simulink library "Batteries"  (R2024b)
settings: Solver=VariableStepAuto  StartTime=0.0  StopTime=10.0  RelTol=1e-3
undefined symbols (not defined in the file or in its folder): battery_builder_rtmsupport, gcbh
libraries: nesl_utility x25, Batteries_lib x25
(part 2 of 2)

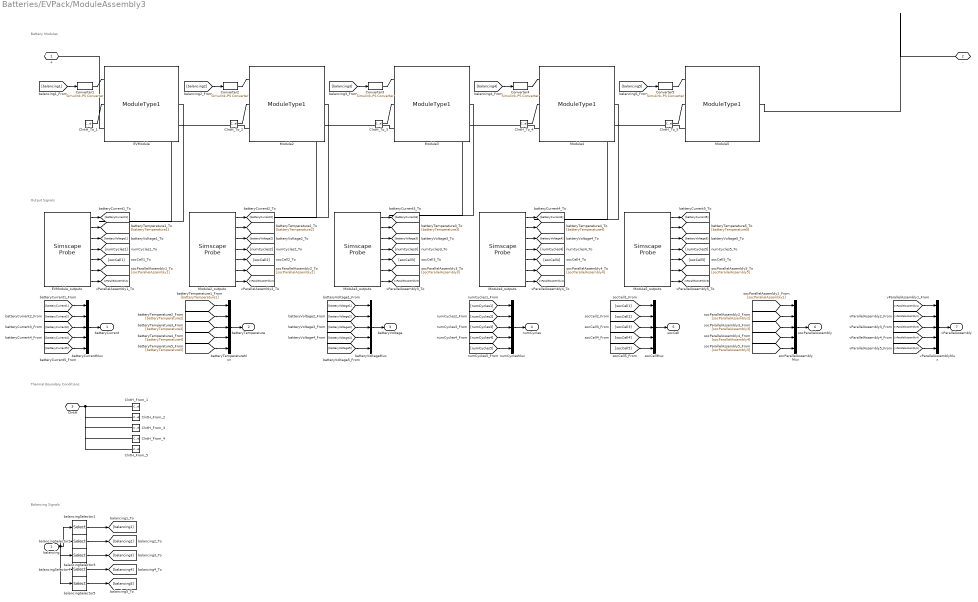
== system Batteries/EVPack/ModuleAssembly3 ==
  note: Balancing Signals
  note: Thermal Boundary Conditions
  note: Output Signals
  note: Battery Modules
  balancing : Inport  PortDimensions=25
  ClntH_From_1 : ConnectionLabel  Label=clntH_1
  ClntH_From_2 : ConnectionLabel  Label=clntH_2
  ClntH_From_3 : ConnectionLabel  Label=clntH_3
  ClntH_From_4 : ConnectionLabel  Label=clntH_4
  ClntH_From_5 : ConnectionLabel  Label=clntH_5
  ClntH_To_1 : ConnectionLabel  Label=clntH_1
  ClntH_To_2 : ConnectionLabel  Label=clntH_2
  ClntH_To_3 : ConnectionLabel  Label=clntH_3
  ClntH_To_4 : ConnectionLabel  Label=clntH_4
  ClntH_To_5 : ConnectionLabel  Label=clntH_5
  Converter{1..5} (5 alike) : nesl_utility/Simulink-PS Converter  PhysicalDomain=network_engine_domain  SubClassName=ps_input  LeftPortType=input  RightPortType=output  PseudoPeriodic=off  Frequencies=[]  NoiseDistribution=none  NoiseParameters=[]  Unit=1  AffineConversion=off  FilteringAndDerivatives=provide  SimscapeFilterOrder=1  InputFilterTimeConstant=0.001  UdotUserProvided=0
  EVModule : Batteries_lib/Modules/ModuleType1  BatteryCapacityCell=27 A*hr  ExtrapolationMethodCell=simscape.enum.extrapolation.nearest  SOCBreakpointsCell=[0, .1, .25, .5, .75, .9, 1]  TemperatureBreakpointsCell=[278, 293, 313] K  OpenCircuitVoltageThermalCell=[3.49, 3.5, 3.51; 3.55, 3.57, 3.56; 3.62, 3.63, 3.64; 3.71, 3.71, 3.72; 3.91, 3.93, 3.94; 4.07, 4.08, 4.08; 4.19, 4.19, 4.19] V  VoltageRangeCell=[0, inf] V  ResistanceSOCBreakpointsCell=[0, .1, .25, .5, .75, .9, 1]  ResistanceTemperatureBreakpointsCell=[278, 293, 313] K  R0ThermalCell=[.0117, .0085, .009; .011, .0085, .009; .0114, .0087, .0092; .0107, .0082, .0088; .0107, .0083, .0091; .0113, .0085, .0089; .0116, .0085, .0089] Ohm  BatteryThermalMassCell=100 J/K  CoolantResistance=1.2 K/W  CellBalancingClosedResistance=0.01 Ohm  CellBalancingOpenConductance=1e-8 1/Ohm  CellBalancingThreshold=0.5  CellBalancingResistance=50 Ohm  P=4  S=5  socCell_specify=off  socCell_priority=High  socCell=1  socCell_nominal_specify=off  socCell_nominal_value=1  socCell_nominal_unit=1  numCycles_specify=off  numCycles_priority=High  numCycles=0  numCycles_nominal_specify=off  numCycles_nominal_value=1  numCycles_nominal_unit=1  batteryVoltage_specify=off  batteryVoltage_priority=None  batteryVoltage=0 V  batteryVoltage_nominal_specify=off  batteryVoltage_nominal_value=1  batteryVoltage_nominal_unit=V  batteryCurrent_specify=off  batteryCurrent_priority=None  batteryCurrent=0 A  batteryCurrent_nominal_specify=off  batteryCurrent_nominal_value=1  batteryCurrent_nominal_unit=A  batteryTemperature_specify=off  batteryTemperature_priority=High  batteryTemperature=298.15 K  batteryTemperature_nominal_specify=off  batteryTemperature_nominal_value=1  batteryTemperature_nominal_unit=K  vParallelAssembly_specify=off  vParallelAssembly_priority=None  vParallelAssembly=repmat(0, 5, 1) V  vParallelAssembly_nominal_specify=off  vParallelAssembly_nominal_value=1  vParallelAssembly_nominal_unit=V  socParallelAssembly_specify=off  socParallelAssembly_priority=None  socParallelAssembly=repmat(1, 5, 1)  socParallelAssembly_nominal_specify=off  socParallelAssembly_nominal_value=1  socParallelAssembly_nominal_unit=1
      settings: InternalSimscapePortConfiguration="{\"Bottom\":[{\"id\":\"n\",\"label\":\"-\",\"type\":\"foundation.electrical.electrical\"}],\"Left\":[{\"id\":\"enableCellBalancing\",\"label\":\"CB\",\"type\":\"input\"},{\"id\":\"ClntH\",\"label\":\"ClntH\",\"type\":\"foundation.thermal.thermal\"}],\"Right\":[],\"Top\":[{\"id\":\"p\",\"label\":\"+\",\"type\":\"foundation.electrical.electrical\"}]}"
  EVModule_outputs : SimscapeProbe  BoundBlock=419  Variables="{\"batteryCurrent\":{\"Unit\":\"A\",\"PortLabel\":\"batteryCurrent\",\"Probing\":\"ON\"},\"batteryTemperature\":{\"Unit\":\"K\",\"PortLabel\":\"batteryTemperature\",\"Probing\":\"ON\"},\"batteryVoltage\":{\"Unit\":\"V\",\"PortLabel\":\"batteryVoltage\",\"Probing\":\"ON\"},\"numCycles\":{\"Unit\":\"1\",\"PortLabel\":\"numCycles\",\"Probing\":\"ON\"},\"socCell\":{\"Unit\":\"1\",\"PortLabel\":\"socCell\",\"Probing\":\"ON\"},\"socParallelAssembly\":{\"Unit\":\"1\",\"PortLabel\":\"socParallelAssembly\",\"Probing\":\"ON\"},\"vParallelAssembly\":{\"Unit\":\"V\",\"PortLabel\":\"vParallelAssembly\",\"Probing\":\"ON\"}}"
  Module{2..5} (4 alike) : Batteries_lib/Modules/ModuleType1  BatteryCapacityCell=27 A*hr  ExtrapolationMethodCell=simscape.enum.extrapolation.nearest  SOCBreakpointsCell=[0, .1, .25, .5, .75, .9, 1]  TemperatureBreakpointsCell=[278, 293, 313] K  OpenCircuitVoltageThermalCell=[3.49, 3.5, 3.51; 3.55, 3.57, 3.56; 3.62, 3.63, 3.64; 3.71, 3.71, 3.72; 3.91, 3.93, 3.94; 4.07, 4.08, 4.08; 4.19, 4.19, 4.19] V  VoltageRangeCell=[0, inf] V  ResistanceSOCBreakpointsCell=[0, .1, .25, .5, .75, .9, 1]  ResistanceTemperatureBreakpointsCell=[278, 293, 313] K  R0ThermalCell=[.0117, .0085, .009; .011, .0085, .009; .0114, .0087, .0092; .0107, .0082, .0088; .0107, .0083, .0091; .0113, .0085, .0089; .0116, .0085, .0089] Ohm  BatteryThermalMassCell=100 J/K  CoolantResistance=1.2 K/W  CellBalancingClosedResistance=0.01 Ohm  CellBalancingOpenConductance=1e-8 1/Ohm  CellBalancingThreshold=0.5  CellBalancingResistance=50 Ohm  P=4  S=5  socCell_specify=off  socCell_priority=High  socCell=1  socCell_nominal_specify=off  socCell_nominal_value=1  socCell_nominal_unit=1  numCycles_specify=off  numCycles_priority=High  numCycles=0  numCycles_nominal_specify=off  numCycles_nominal_value=1  numCycles_nominal_unit=1  batteryVoltage_specify=off  batteryVoltage_priority=None  batteryVoltage=0 V  batteryVoltage_nominal_specify=off  batteryVoltage_nominal_value=1  batteryVoltage_nominal_unit=V  batteryCurrent_specify=off  batteryCurrent_priority=None  batteryCurrent=0 A  batteryCurrent_nominal_specify=off  batteryCurrent_nominal_value=1  batteryCurrent_nominal_unit=A  batteryTemperature_specify=off  batteryTemperature_priority=High  batteryTemperature=298.15 K  batteryTemperature_nominal_specify=off  batteryTemperature_nominal_value=1  batteryTemperature_nominal_unit=K  vParallelAssembly_specify=off  vParallelAssembly_priority=None  vParallelAssembly=repmat(0, 5, 1) V  vParallelAssembly_nominal_specify=off  vParallelAssembly_nominal_value=1  vParallelAssembly_nominal_unit=V  socParallelAssembly_specify=off  socParallelAssembly_priority=None  socParallelAssembly=repmat(1, 5, 1)  socParallelAssembly_nominal_specify=off  socParallelAssembly_nominal_value=1  socParallelAssembly_nominal_unit=1
      settings: InternalSimscapePortConfiguration="{\"Bottom\":[{\"id\":\"n\",\"label\":\"-\",\"type\":\"foundation.electrical.electrical\"}],\"Left\":[{\"id\":\"enableCellBalancing\",\"label\":\"CB\",\"type\":\"input\"},{\"id\":\"ClntH\",\"label\":\"ClntH\",\"type\":\"foundation.thermal.thermal\"}],\"Right\":[],\"Top\":[{\"id\":\"p\",\"label\":\"+\",\"type\":\"foundation.electrical.electrical\"}]}"
  Module2_outputs : SimscapeProbe  BoundBlock=421  Variables="{\"batteryCurrent\":{\"Unit\":\"A\",\"PortLabel\":\"batteryCurrent\",\"Probing\":\"ON\"},\"batteryTemperature\":{\"Unit\":\"K\",\"PortLabel\":\"batteryTemperature\",\"Probing\":\"ON\"},\"batteryVoltage\":{\"Unit\":\"V\",\"PortLabel\":\"batteryVoltage\",\"Probing\":\"ON\"},\"numCycles\":{\"Unit\":\"1\",\"PortLabel\":\"numCycles\",\"Probing\":\"ON\"},\"socCell\":{\"Unit\":\"1\",\"PortLabel\":\"socCell\",\"Probing\":\"ON\"},\"socParallelAssembly\":{\"Unit\":\"1\",\"PortLabel\":\"socParallelAssembly\",\"Probing\":\"ON\"},\"vParallelAssembly\":{\"Unit\":\"V\",\"PortLabel\":\"vParallelAssembly\",\"Probing\":\"ON\"}}"
  Module3_outputs : SimscapeProbe  BoundBlock=423  Variables="{\"batteryCurrent\":{\"Unit\":\"A\",\"PortLabel\":\"batteryCurrent\",\"Probing\":\"ON\"},\"batteryTemperature\":{\"Unit\":\"K\",\"PortLabel\":\"batteryTemperature\",\"Probing\":\"ON\"},\"batteryVoltage\":{\"Unit\":\"V\",\"PortLabel\":\"batteryVoltage\",\"Probing\":\"ON\"},\"numCycles\":{\"Unit\":\"1\",\"PortLabel\":\"numCycles\",\"Probing\":\"ON\"},\"socCell\":{\"Unit\":\"1\",\"PortLabel\":\"socCell\",\"Probing\":\"ON\"},\"socParallelAssembly\":{\"Unit\":\"1\",\"PortLabel\":\"socParallelAssembly\",\"Probing\":\"ON\"},\"vParallelAssembly\":{\"Unit\":\"V\",\"PortLabel\":\"vParallelAssembly\",\"Probing\":\"ON\"}}"
  Module4_outputs : SimscapeProbe  BoundBlock=425  Variables="{\"batteryCurrent\":{\"Unit\":\"A\",\"PortLabel\":\"batteryCurrent\",\"Probing\":\"ON\"},\"batteryTemperature\":{\"Unit\":\"K\",\"PortLabel\":\"batteryTemperature\",\"Probing\":\"ON\"},\"batteryVoltage\":{\"Unit\":\"V\",\"PortLabel\":\"batteryVoltage\",\"Probing\":\"ON\"},\"numCycles\":{\"Unit\":\"1\",\"PortLabel\":\"numCycles\",\"Probing\":\"ON\"},\"socCell\":{\"Unit\":\"1\",\"PortLabel\":\"socCell\",\"Probing\":\"ON\"},\"socParallelAssembly\":{\"Unit\":\"1\",\"PortLabel\":\"socParallelAssembly\",\"Probing\":\"ON\"},\"vParallelAssembly\":{\"Unit\":\"V\",\"PortLabel\":\"vParallelAssembly\",\"Probing\":\"ON\"}}"
  Module5_outputs : SimscapeProbe  BoundBlock=427  Variables="{\"batteryCurrent\":{\"Unit\":\"A\",\"PortLabel\":\"batteryCurrent\",\"Probing\":\"ON\"},\"batteryTemperature\":{\"Unit\":\"K\",\"PortLabel\":\"batteryTemperature\",\"Probing\":\"ON\"},\"batteryVoltage\":{\"Unit\":\"V\",\"PortLabel\":\"batteryVoltage\",\"Probing\":\"ON\"},\"numCycles\":{\"Unit\":\"1\",\"PortLabel\":\"numCycles\",\"Probing\":\"ON\"},\"socCell\":{\"Unit\":\"1\",\"PortLabel\":\"socCell\",\"Probing\":\"ON\"},\"socParallelAssembly\":{\"Unit\":\"1\",\"PortLabel\":\"socParallelAssembly\",\"Probing\":\"ON\"},\"vParallelAssembly\":{\"Unit\":\"V\",\"PortLabel\":\"vParallelAssembly\",\"Probing\":\"ON\"}}"
  balancingSelector1 : Selector  InputPortWidth=25  IndexOptions=Index vector (dialog)  Indices="[1  2  3  4  5]"  OutputSizes=1
  balancingSelector2 : Selector  InputPortWidth=25  IndexOptions=Index vector (dialog)  Indices="[6   7   8   9  10]"  OutputSizes=1
  balancingSelector3 : Selector  InputPortWidth=25  IndexOptions=Index vector (dialog)  Indices="[11  12  13  14  15]"  OutputSizes=1
  balancingSelector4 : Selector  InputPortWidth=25  IndexOptions=Index vector (dialog)  Indices="[16  17  18  19  20]"  OutputSizes=1
  balancingSelector5 : Selector  InputPortWidth=25  IndexOptions=Index vector (dialog)  Indices="[21  22  23  24  25]"  OutputSizes=1
  batteryCurrentMux : Mux  Inputs=5
  batteryTemperatureMux : Mux  Inputs=5
  batteryVoltageMux : Mux  Inputs=5
  numCyclesMux : Mux  Inputs=5
  socCellMux : Mux  Inputs=5
  socParallelAssemblyMux : Mux  Inputs=5
  vParallelAssemblyMux : Mux  Inputs=5
  + : PMIOPort  Side=Left
  - : PMIOPort  Port=2  Side=Right
  ClntH : PMIOPort  Port=3  Side=Right  ConnectionType=Connection: foundation.thermal.thermal
  batteryCurrent : Outport
  batteryTemperature : Outport  Port=2
  batteryVoltage : Outport  Port=3
  numCycles : Outport  Port=4
  socCell : Outport  Port=5
  socParallelAssembly : Outport  Port=6
  vParallelAssembly : Outport  Port=7
  wires:
  balancingSelector5/1 -> [balancing5]
  [balancing5] -> Converter5/1
  balancingSelector4/1 -> [balancing4]
  [balancing4] -> Converter4/1
  balancingSelector3/1 -> [balancing3]
  [balancing3] -> Converter3/1
  balancingSelector2/1 -> [balancing2]
  [balancing2] -> Converter2/1
  balancingSelector1/1 -> [balancing1]
  balancing/1 -> balancingSelector5/1, balancingSelector4/1, balancingSelector3/1, balancingSelector2/1, balancingSelector1/1
  [balancing1] -> Converter1/1
  [vParallelAssembly5] -> vParallelAssemblyMux/5
  Module5_outputs/7 -> [vParallelAssembly5]
  [socParallelAssembly5] -> socParallelAssemblyMux/5
  Module5_outputs/6 -> [socParallelAssembly5]
  [socCell5] -> socCellMux/5
  Module5_outputs/5 -> [socCell5]
  [numCycles5] -> numCyclesMux/5
  Module5_outputs/4 -> [numCycles5]
  [batteryVoltage5] -> batteryVoltageMux/5
  Module5_outputs/3 -> [batteryVoltage5]
  [batteryTemperature5] -> batteryTemperatureMux/5
  Module5_outputs/2 -> [batteryTemperature5]
  [batteryCurrent5] -> batteryCurrentMux/5
  Module5_outputs/1 -> [batteryCurrent5]
  [vParallelAssembly4] -> vParallelAssemblyMux/4
  Module4_outputs/7 -> [vParallelAssembly4]
  [socParallelAssembly4] -> socParallelAssemblyMux/4
  Module4_outputs/6 -> [socParallelAssembly4]
  [socCell4] -> socCellMux/4
  Module4_outputs/5 -> [socCell4]
  [numCycles4] -> numCyclesMux/4
  Module4_outputs/4 -> [numCycles4]
  [batteryVoltage4] -> batteryVoltageMux/4
  Module4_outputs/3 -> [batteryVoltage4]
  [batteryTemperature4] -> batteryTemperatureMux/4
  Module4_outputs/2 -> [batteryTemperature4]
  [batteryCurrent4] -> batteryCurrentMux/4
  Module4_outputs/1 -> [batteryCurrent4]
  [vParallelAssembly3] -> vParallelAssemblyMux/3
  Module3_outputs/7 -> [vParallelAssembly3]
  [socParallelAssembly3] -> socParallelAssemblyMux/3
  Module3_outputs/6 -> [socParallelAssembly3]
  [socCell3] -> socCellMux/3
  Module3_outputs/5 -> [socCell3]
  [numCycles3] -> numCyclesMux/3
  Module3_outputs/4 -> [numCycles3]
  [batteryVoltage3] -> batteryVoltageMux/3
  Module3_outputs/3 -> [batteryVoltage3]
  [batteryTemperature3] -> batteryTemperatureMux/3
  Module3_outputs/2 -> [batteryTemperature3]
  [batteryCurrent3] -> batteryCurrentMux/3
  Module3_outputs/1 -> [batteryCurrent3]
  [vParallelAssembly2] -> vParallelAssemblyMux/2
  Module2_outputs/7 -> [vParallelAssembly2]
  [socParallelAssembly2] -> socParallelAssemblyMux/2
  Module2_outputs/6 -> [socParallelAssembly2]
  [socCell2] -> socCellMux/2
  Module2_outputs/5 -> [socCell2]
  [numCycles2] -> numCyclesMux/2
  Module2_outputs/4 -> [numCycles2]
  [batteryVoltage2] -> batteryVoltageMux/2
  Module2_outputs/3 -> [batteryVoltage2]
  [batteryTemperature2] -> batteryTemperatureMux/2
  Module2_outputs/2 -> [batteryTemperature2]
  [batteryCurrent2] -> batteryCurrentMux/2
  Module2_outputs/1 -> [batteryCurrent2]
  [vParallelAssembly1] -> vParallelAssemblyMux/1
  vParallelAssemblyMux/1 -> vParallelAssembly/1
  EVModule_outputs/7 -> [vParallelAssembly1]
  [socParallelAssembly1] -> socParallelAssemblyMux/1
  socParallelAssemblyMux/1 -> socParallelAssembly/1
  EVModule_outputs/6 -> [socParallelAssembly1]
  [socCell1] -> socCellMux/1
  socCellMux/1 -> socCell/1
  EVModule_outputs/5 -> [socCell1]
  [numCycles1] -> numCyclesMux/1
  numCyclesMux/1 -> numCycles/1
  EVModule_outputs/4 -> [numCycles1]
  [batteryVoltage1] -> batteryVoltageMux/1
  batteryVoltageMux/1 -> batteryVoltage/1
  EVModule_outputs/3 -> [batteryVoltage1]
  [batteryTemperature1] -> batteryTemperatureMux/1
  batteryTemperatureMux/1 -> batteryTemperature/1
  EVModule_outputs/2 -> [batteryTemperature1]
  [batteryCurrent1] -> batteryCurrentMux/1
  batteryCurrentMux/1 -> batteryCurrent/1
  EVModule_outputs/1 -> [batteryCurrent1]
  connections:
  ClntH_To_5/LConn1 -- Module5/LConn2
  ClntH_To_4/LConn1 -- Module4/LConn2
  ClntH_To_3/LConn1 -- Module3/LConn2
  ClntH_To_2/LConn1 -- Module2/LConn2
  ClntH_From_5/LConn1 -- ClntH/RConn1 -- ClntH_From_4/LConn1 -- ClntH_From_3/LConn1 -- ClntH_From_2/LConn1 -- ClntH_From_1/LConn1
  ClntH_To_1/LConn1 -- EVModule/LConn2
  Converter5/RConn1 -- Module5/LConn1
  Converter4/RConn1 -- Module4/LConn1
  Converter3/RConn1 -- Module3/LConn1
  Converter2/RConn1 -- Module2/LConn1
  Converter1/RConn1 -- EVModule/LConn1
  Module5/RConn1 -- -/RConn1
  EVModule/LConn3 -- +/RConn1
  Module5/LConn3 -- Module4/RConn1
  Module4/LConn3 -- Module3/RConn1
  Module3/LConn3 -- Module2/RConn1
  Module2/LConn3 -- EVModule/RConn1

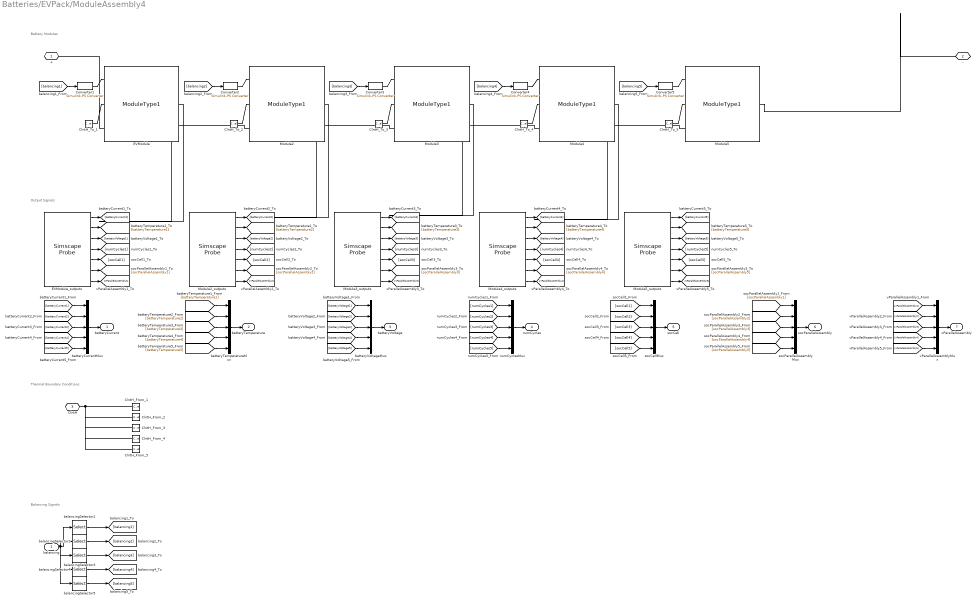
== system Batteries/EVPack/ModuleAssembly4 ==
  note: Balancing Signals
  note: Thermal Boundary Conditions
  note: Output Signals
  note: Battery Modules
  balancing : Inport  PortDimensions=25
  ClntH_From_1 : ConnectionLabel  Label=clntH_1
  ClntH_From_2 : ConnectionLabel  Label=clntH_2
  ClntH_From_3 : ConnectionLabel  Label=clntH_3
  ClntH_From_4 : ConnectionLabel  Label=clntH_4
  ClntH_From_5 : ConnectionLabel  Label=clntH_5
  ClntH_To_1 : ConnectionLabel  Label=clntH_1
  ClntH_To_2 : ConnectionLabel  Label=clntH_2
  ClntH_To_3 : ConnectionLabel  Label=clntH_3
  ClntH_To_4 : ConnectionLabel  Label=clntH_4
  ClntH_To_5 : ConnectionLabel  Label=clntH_5
  Converter{1..5} (5 alike) : nesl_utility/Simulink-PS Converter  PhysicalDomain=network_engine_domain  SubClassName=ps_input  LeftPortType=input  RightPortType=output  PseudoPeriodic=off  Frequencies=[]  NoiseDistribution=none  NoiseParameters=[]  Unit=1  AffineConversion=off  FilteringAndDerivatives=provide  SimscapeFilterOrder=1  InputFilterTimeConstant=0.001  UdotUserProvided=0
  EVModule : Batteries_lib/Modules/ModuleType1  BatteryCapacityCell=27 A*hr  ExtrapolationMethodCell=simscape.enum.extrapolation.nearest  SOCBreakpointsCell=[0, .1, .25, .5, .75, .9, 1]  TemperatureBreakpointsCell=[278, 293, 313] K  OpenCircuitVoltageThermalCell=[3.49, 3.5, 3.51; 3.55, 3.57, 3.56; 3.62, 3.63, 3.64; 3.71, 3.71, 3.72; 3.91, 3.93, 3.94; 4.07, 4.08, 4.08; 4.19, 4.19, 4.19] V  VoltageRangeCell=[0, inf] V  ResistanceSOCBreakpointsCell=[0, .1, .25, .5, .75, .9, 1]  ResistanceTemperatureBreakpointsCell=[278, 293, 313] K  R0ThermalCell=[.0117, .0085, .009; .011, .0085, .009; .0114, .0087, .0092; .0107, .0082, .0088; .0107, .0083, .0091; .0113, .0085, .0089; .0116, .0085, .0089] Ohm  BatteryThermalMassCell=100 J/K  CoolantResistance=1.2 K/W  CellBalancingClosedResistance=0.01 Ohm  CellBalancingOpenConductance=1e-8 1/Ohm  CellBalancingThreshold=0.5  CellBalancingResistance=50 Ohm  P=4  S=5  socCell_specify=off  socCell_priority=High  socCell=1  socCell_nominal_specify=off  socCell_nominal_value=1  socCell_nominal_unit=1  numCycles_specify=off  numCycles_priority=High  numCycles=0  numCycles_nominal_specify=off  numCycles_nominal_value=1  numCycles_nominal_unit=1  batteryVoltage_specify=off  batteryVoltage_priority=None  batteryVoltage=0 V  batteryVoltage_nominal_specify=off  batteryVoltage_nominal_value=1  batteryVoltage_nominal_unit=V  batteryCurrent_specify=off  batteryCurrent_priority=None  batteryCurrent=0 A  batteryCurrent_nominal_specify=off  batteryCurrent_nominal_value=1  batteryCurrent_nominal_unit=A  batteryTemperature_specify=off  batteryTemperature_priority=High  batteryTemperature=298.15 K  batteryTemperature_nominal_specify=off  batteryTemperature_nominal_value=1  batteryTemperature_nominal_unit=K  vParallelAssembly_specify=off  vParallelAssembly_priority=None  vParallelAssembly=repmat(0, 5, 1) V  vParallelAssembly_nominal_specify=off  vParallelAssembly_nominal_value=1  vParallelAssembly_nominal_unit=V  socParallelAssembly_specify=off  socParallelAssembly_priority=None  socParallelAssembly=repmat(1, 5, 1)  socParallelAssembly_nominal_specify=off  socParallelAssembly_nominal_value=1  socParallelAssembly_nominal_unit=1
      settings: InternalSimscapePortConfiguration="{\"Bottom\":[{\"id\":\"n\",\"label\":\"-\",\"type\":\"foundation.electrical.electrical\"}],\"Left\":[{\"id\":\"enableCellBalancing\",\"label\":\"CB\",\"type\":\"input\"},{\"id\":\"ClntH\",\"label\":\"ClntH\",\"type\":\"foundation.thermal.thermal\"}],\"Right\":[],\"Top\":[{\"id\":\"p\",\"label\":\"+\",\"type\":\"foundation.electrical.electrical\"}]}"
  EVModule_outputs : SimscapeProbe  BoundBlock=552  Variables="{\"batteryCurrent\":{\"Unit\":\"A\",\"PortLabel\":\"batteryCurrent\",\"Probing\":\"ON\"},\"batteryTemperature\":{\"Unit\":\"K\",\"PortLabel\":\"batteryTemperature\",\"Probing\":\"ON\"},\"batteryVoltage\":{\"Unit\":\"V\",\"PortLabel\":\"batteryVoltage\",\"Probing\":\"ON\"},\"numCycles\":{\"Unit\":\"1\",\"PortLabel\":\"numCycles\",\"Probing\":\"ON\"},\"socCell\":{\"Unit\":\"1\",\"PortLabel\":\"socCell\",\"Probing\":\"ON\"},\"socParallelAssembly\":{\"Unit\":\"1\",\"PortLabel\":\"socParallelAssembly\",\"Probing\":\"ON\"},\"vParallelAssembly\":{\"Unit\":\"V\",\"PortLabel\":\"vParallelAssembly\",\"Probing\":\"ON\"}}"
  Module{2..5} (4 alike) : Batteries_lib/Modules/ModuleType1  BatteryCapacityCell=27 A*hr  ExtrapolationMethodCell=simscape.enum.extrapolation.nearest  SOCBreakpointsCell=[0, .1, .25, .5, .75, .9, 1]  TemperatureBreakpointsCell=[278, 293, 313] K  OpenCircuitVoltageThermalCell=[3.49, 3.5, 3.51; 3.55, 3.57, 3.56; 3.62, 3.63, 3.64; 3.71, 3.71, 3.72; 3.91, 3.93, 3.94; 4.07, 4.08, 4.08; 4.19, 4.19, 4.19] V  VoltageRangeCell=[0, inf] V  ResistanceSOCBreakpointsCell=[0, .1, .25, .5, .75, .9, 1]  ResistanceTemperatureBreakpointsCell=[278, 293, 313] K  R0ThermalCell=[.0117, .0085, .009; .011, .0085, .009; .0114, .0087, .0092; .0107, .0082, .0088; .0107, .0083, .0091; .0113, .0085, .0089; .0116, .0085, .0089] Ohm  BatteryThermalMassCell=100 J/K  CoolantResistance=1.2 K/W  CellBalancingClosedResistance=0.01 Ohm  CellBalancingOpenConductance=1e-8 1/Ohm  CellBalancingThreshold=0.5  CellBalancingResistance=50 Ohm  P=4  S=5  socCell_specify=off  socCell_priority=High  socCell=1  socCell_nominal_specify=off  socCell_nominal_value=1  socCell_nominal_unit=1  numCycles_specify=off  numCycles_priority=High  numCycles=0  numCycles_nominal_specify=off  numCycles_nominal_value=1  numCycles_nominal_unit=1  batteryVoltage_specify=off  batteryVoltage_priority=None  batteryVoltage=0 V  batteryVoltage_nominal_specify=off  batteryVoltage_nominal_value=1  batteryVoltage_nominal_unit=V  batteryCurrent_specify=off  batteryCurrent_priority=None  batteryCurrent=0 A  batteryCurrent_nominal_specify=off  batteryCurrent_nominal_value=1  batteryCurrent_nominal_unit=A  batteryTemperature_specify=off  batteryTemperature_priority=High  batteryTemperature=298.15 K  batteryTemperature_nominal_specify=off  batteryTemperature_nominal_value=1  batteryTemperature_nominal_unit=K  vParallelAssembly_specify=off  vParallelAssembly_priority=None  vParallelAssembly=repmat(0, 5, 1) V  vParallelAssembly_nominal_specify=off  vParallelAssembly_nominal_value=1  vParallelAssembly_nominal_unit=V  socParallelAssembly_specify=off  socParallelAssembly_priority=None  socParallelAssembly=repmat(1, 5, 1)  socParallelAssembly_nominal_specify=off  socParallelAssembly_nominal_value=1  socParallelAssembly_nominal_unit=1
      settings: InternalSimscapePortConfiguration="{\"Bottom\":[{\"id\":\"n\",\"label\":\"-\",\"type\":\"foundation.electrical.electrical\"}],\"Left\":[{\"id\":\"enableCellBalancing\",\"label\":\"CB\",\"type\":\"input\"},{\"id\":\"ClntH\",\"label\":\"ClntH\",\"type\":\"foundation.thermal.thermal\"}],\"Right\":[],\"Top\":[{\"id\":\"p\",\"label\":\"+\",\"type\":\"foundation.electrical.electrical\"}]}"
  Module2_outputs : SimscapeProbe  BoundBlock=554  Variables="{\"batteryCurrent\":{\"Unit\":\"A\",\"PortLabel\":\"batteryCurrent\",\"Probing\":\"ON\"},\"batteryTemperature\":{\"Unit\":\"K\",\"PortLabel\":\"batteryTemperature\",\"Probing\":\"ON\"},\"batteryVoltage\":{\"Unit\":\"V\",\"PortLabel\":\"batteryVoltage\",\"Probing\":\"ON\"},\"numCycles\":{\"Unit\":\"1\",\"PortLabel\":\"numCycles\",\"Probing\":\"ON\"},\"socCell\":{\"Unit\":\"1\",\"PortLabel\":\"socCell\",\"Probing\":\"ON\"},\"socParallelAssembly\":{\"Unit\":\"1\",\"PortLabel\":\"socParallelAssembly\",\"Probing\":\"ON\"},\"vParallelAssembly\":{\"Unit\":\"V\",\"PortLabel\":\"vParallelAssembly\",\"Probing\":\"ON\"}}"
  Module3_outputs : SimscapeProbe  BoundBlock=556  Variables="{\"batteryCurrent\":{\"Unit\":\"A\",\"PortLabel\":\"batteryCurrent\",\"Probing\":\"ON\"},\"batteryTemperature\":{\"Unit\":\"K\",\"PortLabel\":\"batteryTemperature\",\"Probing\":\"ON\"},\"batteryVoltage\":{\"Unit\":\"V\",\"PortLabel\":\"batteryVoltage\",\"Probing\":\"ON\"},\"numCycles\":{\"Unit\":\"1\",\"PortLabel\":\"numCycles\",\"Probing\":\"ON\"},\"socCell\":{\"Unit\":\"1\",\"PortLabel\":\"socCell\",\"Probing\":\"ON\"},\"socParallelAssembly\":{\"Unit\":\"1\",\"PortLabel\":\"socParallelAssembly\",\"Probing\":\"ON\"},\"vParallelAssembly\":{\"Unit\":\"V\",\"PortLabel\":\"vParallelAssembly\",\"Probing\":\"ON\"}}"
  Module4_outputs : SimscapeProbe  BoundBlock=558  Variables="{\"batteryCurrent\":{\"Unit\":\"A\",\"PortLabel\":\"batteryCurrent\",\"Probing\":\"ON\"},\"batteryTemperature\":{\"Unit\":\"K\",\"PortLabel\":\"batteryTemperature\",\"Probing\":\"ON\"},\"batteryVoltage\":{\"Unit\":\"V\",\"PortLabel\":\"batteryVoltage\",\"Probing\":\"ON\"},\"numCycles\":{\"Unit\":\"1\",\"PortLabel\":\"numCycles\",\"Probing\":\"ON\"},\"socCell\":{\"Unit\":\"1\",\"PortLabel\":\"socCell\",\"Probing\":\"ON\"},\"socParallelAssembly\":{\"Unit\":\"1\",\"PortLabel\":\"socParallelAssembly\",\"Probing\":\"ON\"},\"vParallelAssembly\":{\"Unit\":\"V\",\"PortLabel\":\"vParallelAssembly\",\"Probing\":\"ON\"}}"
  Module5_outputs : SimscapeProbe  BoundBlock=560  Variables="{\"batteryCurrent\":{\"Unit\":\"A\",\"PortLabel\":\"batteryCurrent\",\"Probing\":\"ON\"},\"batteryTemperature\":{\"Unit\":\"K\",\"PortLabel\":\"batteryTemperature\",\"Probing\":\"ON\"},\"batteryVoltage\":{\"Unit\":\"V\",\"PortLabel\":\"batteryVoltage\",\"Probing\":\"ON\"},\"numCycles\":{\"Unit\":\"1\",\"PortLabel\":\"numCycles\",\"Probing\":\"ON\"},\"socCell\":{\"Unit\":\"1\",\"PortLabel\":\"socCell\",\"Probing\":\"ON\"},\"socParallelAssembly\":{\"Unit\":\"1\",\"PortLabel\":\"socParallelAssembly\",\"Probing\":\"ON\"},\"vParallelAssembly\":{\"Unit\":\"V\",\"PortLabel\":\"vParallelAssembly\",\"Probing\":\"ON\"}}"
  balancingSelector1 : Selector  InputPortWidth=25  IndexOptions=Index vector (dialog)  Indices="[1  2  3  4  5]"  OutputSizes=1
  balancingSelector2 : Selector  InputPortWidth=25  IndexOptions=Index vector (dialog)  Indices="[6   7   8   9  10]"  OutputSizes=1
  balancingSelector3 : Selector  InputPortWidth=25  IndexOptions=Index vector (dialog)  Indices="[11  12  13  14  15]"  OutputSizes=1
  balancingSelector4 : Selector  InputPortWidth=25  IndexOptions=Index vector (dialog)  Indices="[16  17  18  19  20]"  OutputSizes=1
  balancingSelector5 : Selector  InputPortWidth=25  IndexOptions=Index vector (dialog)  Indices="[21  22  23  24  25]"  OutputSizes=1
  batteryCurrentMux : Mux  Inputs=5
  batteryTemperatureMux : Mux  Inputs=5
  batteryVoltageMux : Mux  Inputs=5
  numCyclesMux : Mux  Inputs=5
  socCellMux : Mux  Inputs=5
  socParallelAssemblyMux : Mux  Inputs=5
  vParallelAssemblyMux : Mux  Inputs=5
  + : PMIOPort  Side=Left
  - : PMIOPort  Port=2  Side=Right
  ClntH : PMIOPort  Port=3  Side=Right  ConnectionType=Connection: foundation.thermal.thermal
  batteryCurrent : Outport
  batteryTemperature : Outport  Port=2
  batteryVoltage : Outport  Port=3
  numCycles : Outport  Port=4
  socCell : Outport  Port=5
  socParallelAssembly : Outport  Port=6
  vParallelAssembly : Outport  Port=7
  wires:
  balancingSelector5/1 -> [balancing5]
  [balancing5] -> Converter5/1
  balancingSelector4/1 -> [balancing4]
  [balancing4] -> Converter4/1
  balancingSelector3/1 -> [balancing3]
  [balancing3] -> Converter3/1
  balancingSelector2/1 -> [balancing2]
  [balancing2] -> Converter2/1
  balancingSelector1/1 -> [balancing1]
  balancing/1 -> balancingSelector5/1, balancingSelector4/1, balancingSelector3/1, balancingSelector2/1, balancingSelector1/1
  [balancing1] -> Converter1/1
  [vParallelAssembly5] -> vParallelAssemblyMux/5
  Module5_outputs/7 -> [vParallelAssembly5]
  [socParallelAssembly5] -> socParallelAssemblyMux/5
  Module5_outputs/6 -> [socParallelAssembly5]
  [socCell5] -> socCellMux/5
  Module5_outputs/5 -> [socCell5]
  [numCycles5] -> numCyclesMux/5
  Module5_outputs/4 -> [numCycles5]
  [batteryVoltage5] -> batteryVoltageMux/5
  Module5_outputs/3 -> [batteryVoltage5]
  [batteryTemperature5] -> batteryTemperatureMux/5
  Module5_outputs/2 -> [batteryTemperature5]
  [batteryCurrent5] -> batteryCurrentMux/5
  Module5_outputs/1 -> [batteryCurrent5]
  [vParallelAssembly4] -> vParallelAssemblyMux/4
  Module4_outputs/7 -> [vParallelAssembly4]
  [socParallelAssembly4] -> socParallelAssemblyMux/4
  Module4_outputs/6 -> [socParallelAssembly4]
  [socCell4] -> socCellMux/4
  Module4_outputs/5 -> [socCell4]
  [numCycles4] -> numCyclesMux/4
  Module4_outputs/4 -> [numCycles4]
  [batteryVoltage4] -> batteryVoltageMux/4
  Module4_outputs/3 -> [batteryVoltage4]
  [batteryTemperature4] -> batteryTemperatureMux/4
  Module4_outputs/2 -> [batteryTemperature4]
  [batteryCurrent4] -> batteryCurrentMux/4
  Module4_outputs/1 -> [batteryCurrent4]
  [vParallelAssembly3] -> vParallelAssemblyMux/3
  Module3_outputs/7 -> [vParallelAssembly3]
  [socParallelAssembly3] -> socParallelAssemblyMux/3
  Module3_outputs/6 -> [socParallelAssembly3]
  [socCell3] -> socCellMux/3
  Module3_outputs/5 -> [socCell3]
  [numCycles3] -> numCyclesMux/3
  Module3_outputs/4 -> [numCycles3]
  [batteryVoltage3] -> batteryVoltageMux/3
  Module3_outputs/3 -> [batteryVoltage3]
  [batteryTemperature3] -> batteryTemperatureMux/3
  Module3_outputs/2 -> [batteryTemperature3]
  [batteryCurrent3] -> batteryCurrentMux/3
  Module3_outputs/1 -> [batteryCurrent3]
  [vParallelAssembly2] -> vParallelAssemblyMux/2
  Module2_outputs/7 -> [vParallelAssembly2]
  [socParallelAssembly2] -> socParallelAssemblyMux/2
  Module2_outputs/6 -> [socParallelAssembly2]
  [socCell2] -> socCellMux/2
  Module2_outputs/5 -> [socCell2]
  [numCycles2] -> numCyclesMux/2
  Module2_outputs/4 -> [numCycles2]
  [batteryVoltage2] -> batteryVoltageMux/2
  Module2_outputs/3 -> [batteryVoltage2]
  [batteryTemperature2] -> batteryTemperatureMux/2
  Module2_outputs/2 -> [batteryTemperature2]
  [batteryCurrent2] -> batteryCurrentMux/2
  Module2_outputs/1 -> [batteryCurrent2]
  [vParallelAssembly1] -> vParallelAssemblyMux/1
  vParallelAssemblyMux/1 -> vParallelAssembly/1
  EVModule_outputs/7 -> [vParallelAssembly1]
  [socParallelAssembly1] -> socParallelAssemblyMux/1
  socParallelAssemblyMux/1 -> socParallelAssembly/1
  EVModule_outputs/6 -> [socParallelAssembly1]
  [socCell1] -> socCellMux/1
  socCellMux/1 -> socCell/1
  EVModule_outputs/5 -> [socCell1]
  [numCycles1] -> numCyclesMux/1
  numCyclesMux/1 -> numCycles/1
  EVModule_outputs/4 -> [numCycles1]
  [batteryVoltage1] -> batteryVoltageMux/1
  batteryVoltageMux/1 -> batteryVoltage/1
  EVModule_outputs/3 -> [batteryVoltage1]
  [batteryTemperature1] -> batteryTemperatureMux/1
  batteryTemperatureMux/1 -> batteryTemperature/1
  EVModule_outputs/2 -> [batteryTemperature1]
  [batteryCurrent1] -> batteryCurrentMux/1
  batteryCurrentMux/1 -> batteryCurrent/1
  EVModule_outputs/1 -> [batteryCurrent1]
  connections:
  ClntH_To_5/LConn1 -- Module5/LConn2
  ClntH_To_4/LConn1 -- Module4/LConn2
  ClntH_To_3/LConn1 -- Module3/LConn2
  ClntH_To_2/LConn1 -- Module2/LConn2
  ClntH_From_5/LConn1 -- ClntH/RConn1 -- ClntH_From_4/LConn1 -- ClntH_From_3/LConn1 -- ClntH_From_2/LConn1 -- ClntH_From_1/LConn1
  ClntH_To_1/LConn1 -- EVModule/LConn2
  Converter5/RConn1 -- Module5/LConn1
  Converter4/RConn1 -- Module4/LConn1
  Converter3/RConn1 -- Module3/LConn1
  Converter2/RConn1 -- Module2/LConn1
  Converter1/RConn1 -- EVModule/LConn1
  Module5/RConn1 -- -/RConn1
  EVModule/LConn3 -- +/RConn1
  Module5/LConn3 -- Module4/RConn1
  Module4/LConn3 -- Module3/RConn1
  Module3/LConn3 -- Module2/RConn1
  Module2/LConn3 -- EVModule/RConn1

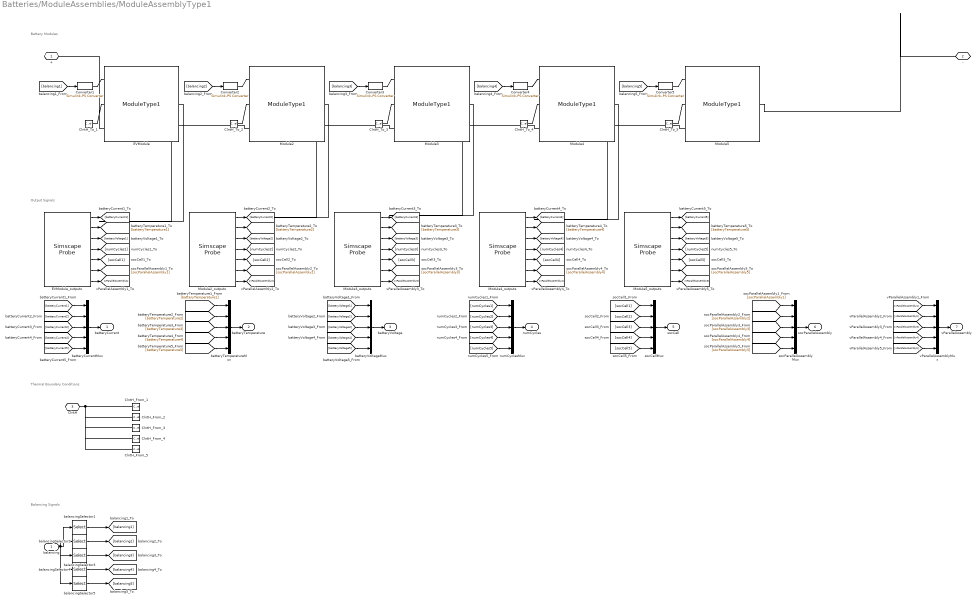
== system Batteries/ModuleAssemblies/ModuleAssemblyType1 ==
  note: Battery Modules
  note: Output Signals
  note: Thermal Boundary Conditions
  note: Balancing Signals
  balancing : Inport  PortDimensions=25
  ClntH_From_1 : ConnectionLabel  Label=clntH_1
  ClntH_From_2 : ConnectionLabel  Label=clntH_2
  ClntH_From_3 : ConnectionLabel  Label=clntH_3
  ClntH_From_4 : ConnectionLabel  Label=clntH_4
  ClntH_From_5 : ConnectionLabel  Label=clntH_5
  ClntH_To_1 : ConnectionLabel  Label=clntH_1
  ClntH_To_2 : ConnectionLabel  Label=clntH_2
  ClntH_To_3 : ConnectionLabel  Label=clntH_3
  ClntH_To_4 : ConnectionLabel  Label=clntH_4
  ClntH_To_5 : ConnectionLabel  Label=clntH_5
  Converter{1..5} (5 alike) : nesl_utility/Simulink-PS Converter  PhysicalDomain=network_engine_domain  SubClassName=ps_input  LeftPortType=input  RightPortType=output  PseudoPeriodic=off  Frequencies=[]  NoiseDistribution=none  NoiseParameters=[]  Unit=1  AffineConversion=off  FilteringAndDerivatives=provide  SimscapeFilterOrder=1  InputFilterTimeConstant=0.001  UdotUserProvided=0
  EVModule : Batteries_lib/Modules/ModuleType1  BatteryCapacityCell=27 A*hr  ExtrapolationMethodCell=simscape.enum.extrapolation.nearest  SOCBreakpointsCell=[0, .1, .25, .5, .75, .9, 1]  TemperatureBreakpointsCell=[278, 293, 313] K  OpenCircuitVoltageThermalCell=[3.49, 3.5, 3.51; 3.55, 3.57, 3.56; 3.62, 3.63, 3.64; 3.71, 3.71, 3.72; 3.91, 3.93, 3.94; 4.07, 4.08, 4.08; 4.19, 4.19, 4.19] V  VoltageRangeCell=[0, inf] V  ResistanceSOCBreakpointsCell=[0, .1, .25, .5, .75, .9, 1]  ResistanceTemperatureBreakpointsCell=[278, 293, 313] K  R0ThermalCell=[.0117, .0085, .009; .011, .0085, .009; .0114, .0087, .0092; .0107, .0082, .0088; .0107, .0083, .0091; .0113, .0085, .0089; .0116, .0085, .0089] Ohm  BatteryThermalMassCell=100 J/K  CoolantResistance=1.2 K/W  CellBalancingClosedResistance=0.01 Ohm  CellBalancingOpenConductance=1e-8 1/Ohm  CellBalancingThreshold=0.5  CellBalancingResistance=50 Ohm  P=4  S=5  socCell_specify=off  socCell_priority=High  socCell=1  socCell_nominal_specify=off  socCell_nominal_value=1  socCell_nominal_unit=1  numCycles_specify=off  numCycles_priority=High  numCycles=0  numCycles_nominal_specify=off  numCycles_nominal_value=1  numCycles_nominal_unit=1  batteryVoltage_specify=off  batteryVoltage_priority=None  batteryVoltage=0 V  batteryVoltage_nominal_specify=off  batteryVoltage_nominal_value=1  batteryVoltage_nominal_unit=V  batteryCurrent_specify=off  batteryCurrent_priority=None  batteryCurrent=0 A  batteryCurrent_nominal_specify=off  batteryCurrent_nominal_value=1  batteryCurrent_nominal_unit=A  batteryTemperature_specify=off  batteryTemperature_priority=High  batteryTemperature=298.15 K  batteryTemperature_nominal_specify=off  batteryTemperature_nominal_value=1  batteryTemperature_nominal_unit=K  vParallelAssembly_specify=off  vParallelAssembly_priority=None  vParallelAssembly=repmat(0, 5, 1) V  vParallelAssembly_nominal_specify=off  vParallelAssembly_nominal_value=1  vParallelAssembly_nominal_unit=V  socParallelAssembly_specify=off  socParallelAssembly_priority=None  socParallelAssembly=repmat(1, 5, 1)  socParallelAssembly_nominal_specify=off  socParallelAssembly_nominal_value=1  socParallelAssembly_nominal_unit=1
      settings: InternalSimscapePortConfiguration="{\"Bottom\":[{\"id\":\"n\",\"label\":\"-\",\"type\":\"foundation.electrical.electrical\"}],\"Left\":[{\"id\":\"enableCellBalancing\",\"label\":\"CB\",\"type\":\"input\"},{\"id\":\"ClntH\",\"label\":\"ClntH\",\"type\":\"foundation.thermal.thermal\"}],\"Right\":[],\"Top\":[{\"id\":\"p\",\"label\":\"+\",\"type\":\"foundation.electrical.electrical\"}]}"
  EVModule_outputs : SimscapeProbe  BoundBlock=3  Variables="{\"batteryCurrent\":{\"Unit\":\"A\",\"PortLabel\":\"batteryCurrent\",\"Probing\":\"ON\"},\"batteryTemperature\":{\"Unit\":\"K\",\"PortLabel\":\"batteryTemperature\",\"Probing\":\"ON\"},\"batteryVoltage\":{\"Unit\":\"V\",\"PortLabel\":\"batteryVoltage\",\"Probing\":\"ON\"},\"numCycles\":{\"Unit\":\"1\",\"PortLabel\":\"numCycles\",\"Probing\":\"ON\"},\"socCell\":{\"Unit\":\"1\",\"PortLabel\":\"socCell\",\"Probing\":\"ON\"},\"socParallelAssembly\":{\"Unit\":\"1\",\"PortLabel\":\"socParallelAssembly\",\"Probing\":\"ON\"},\"vParallelAssembly\":{\"Unit\":\"V\",\"PortLabel\":\"vParallelAssembly\",\"Probing\":\"ON\"}}"
  Module{2..5} (4 alike) : Batteries_lib/Modules/ModuleType1  BatteryCapacityCell=27 A*hr  ExtrapolationMethodCell=simscape.enum.extrapolation.nearest  SOCBreakpointsCell=[0, .1, .25, .5, .75, .9, 1]  TemperatureBreakpointsCell=[278, 293, 313] K  OpenCircuitVoltageThermalCell=[3.49, 3.5, 3.51; 3.55, 3.57, 3.56; 3.62, 3.63, 3.64; 3.71, 3.71, 3.72; 3.91, 3.93, 3.94; 4.07, 4.08, 4.08; 4.19, 4.19, 4.19] V  VoltageRangeCell=[0, inf] V  ResistanceSOCBreakpointsCell=[0, .1, .25, .5, .75, .9, 1]  ResistanceTemperatureBreakpointsCell=[278, 293, 313] K  R0ThermalCell=[.0117, .0085, .009; .011, .0085, .009; .0114, .0087, .0092; .0107, .0082, .0088; .0107, .0083, .0091; .0113, .0085, .0089; .0116, .0085, .0089] Ohm  BatteryThermalMassCell=100 J/K  CoolantResistance=1.2 K/W  CellBalancingClosedResistance=0.01 Ohm  CellBalancingOpenConductance=1e-8 1/Ohm  CellBalancingThreshold=0.5  CellBalancingResistance=50 Ohm  P=4  S=5  socCell_specify=off  socCell_priority=High  socCell=1  socCell_nominal_specify=off  socCell_nominal_value=1  socCell_nominal_unit=1  numCycles_specify=off  numCycles_priority=High  numCycles=0  numCycles_nominal_specify=off  numCycles_nominal_value=1  numCycles_nominal_unit=1  batteryVoltage_specify=off  batteryVoltage_priority=None  batteryVoltage=0 V  batteryVoltage_nominal_specify=off  batteryVoltage_nominal_value=1  batteryVoltage_nominal_unit=V  batteryCurrent_specify=off  batteryCurrent_priority=None  batteryCurrent=0 A  batteryCurrent_nominal_specify=off  batteryCurrent_nominal_value=1  batteryCurrent_nominal_unit=A  batteryTemperature_specify=off  batteryTemperature_priority=High  batteryTemperature=298.15 K  batteryTemperature_nominal_specify=off  batteryTemperature_nominal_value=1  batteryTemperature_nominal_unit=K  vParallelAssembly_specify=off  vParallelAssembly_priority=None  vParallelAssembly=repmat(0, 5, 1) V  vParallelAssembly_nominal_specify=off  vParallelAssembly_nominal_value=1  vParallelAssembly_nominal_unit=V  socParallelAssembly_specify=off  socParallelAssembly_priority=None  socParallelAssembly=repmat(1, 5, 1)  socParallelAssembly_nominal_specify=off  socParallelAssembly_nominal_value=1  socParallelAssembly_nominal_unit=1
      settings: InternalSimscapePortConfiguration="{\"Bottom\":[{\"id\":\"n\",\"label\":\"-\",\"type\":\"foundation.electrical.electrical\"}],\"Left\":[{\"id\":\"enableCellBalancing\",\"label\":\"CB\",\"type\":\"input\"},{\"id\":\"ClntH\",\"label\":\"ClntH\",\"type\":\"foundation.thermal.thermal\"}],\"Right\":[],\"Top\":[{\"id\":\"p\",\"label\":\"+\",\"type\":\"foundation.electrical.electrical\"}]}"
  Module2_outputs : SimscapeProbe  BoundBlock=4  Variables="{\"batteryCurrent\":{\"Unit\":\"A\",\"PortLabel\":\"batteryCurrent\",\"Probing\":\"ON\"},\"batteryTemperature\":{\"Unit\":\"K\",\"PortLabel\":\"batteryTemperature\",\"Probing\":\"ON\"},\"batteryVoltage\":{\"Unit\":\"V\",\"PortLabel\":\"batteryVoltage\",\"Probing\":\"ON\"},\"numCycles\":{\"Unit\":\"1\",\"PortLabel\":\"numCycles\",\"Probing\":\"ON\"},\"socCell\":{\"Unit\":\"1\",\"PortLabel\":\"socCell\",\"Probing\":\"ON\"},\"socParallelAssembly\":{\"Unit\":\"1\",\"PortLabel\":\"socParallelAssembly\",\"Probing\":\"ON\"},\"vParallelAssembly\":{\"Unit\":\"V\",\"PortLabel\":\"vParallelAssembly\",\"Probing\":\"ON\"}}"
  Module3_outputs : SimscapeProbe  BoundBlock=5  Variables="{\"batteryCurrent\":{\"Unit\":\"A\",\"PortLabel\":\"batteryCurrent\",\"Probing\":\"ON\"},\"batteryTemperature\":{\"Unit\":\"K\",\"PortLabel\":\"batteryTemperature\",\"Probing\":\"ON\"},\"batteryVoltage\":{\"Unit\":\"V\",\"PortLabel\":\"batteryVoltage\",\"Probing\":\"ON\"},\"numCycles\":{\"Unit\":\"1\",\"PortLabel\":\"numCycles\",\"Probing\":\"ON\"},\"socCell\":{\"Unit\":\"1\",\"PortLabel\":\"socCell\",\"Probing\":\"ON\"},\"socParallelAssembly\":{\"Unit\":\"1\",\"PortLabel\":\"socParallelAssembly\",\"Probing\":\"ON\"},\"vParallelAssembly\":{\"Unit\":\"V\",\"PortLabel\":\"vParallelAssembly\",\"Probing\":\"ON\"}}"
  Module4_outputs : SimscapeProbe  BoundBlock=6  Variables="{\"batteryCurrent\":{\"Unit\":\"A\",\"PortLabel\":\"batteryCurrent\",\"Probing\":\"ON\"},\"batteryTemperature\":{\"Unit\":\"K\",\"PortLabel\":\"batteryTemperature\",\"Probing\":\"ON\"},\"batteryVoltage\":{\"Unit\":\"V\",\"PortLabel\":\"batteryVoltage\",\"Probing\":\"ON\"},\"numCycles\":{\"Unit\":\"1\",\"PortLabel\":\"numCycles\",\"Probing\":\"ON\"},\"socCell\":{\"Unit\":\"1\",\"PortLabel\":\"socCell\",\"Probing\":\"ON\"},\"socParallelAssembly\":{\"Unit\":\"1\",\"PortLabel\":\"socParallelAssembly\",\"Probing\":\"ON\"},\"vParallelAssembly\":{\"Unit\":\"V\",\"PortLabel\":\"vParallelAssembly\",\"Probing\":\"ON\"}}"
  Module5_outputs : SimscapeProbe  BoundBlock=7  Variables="{\"batteryCurrent\":{\"Unit\":\"A\",\"PortLabel\":\"batteryCurrent\",\"Probing\":\"ON\"},\"batteryTemperature\":{\"Unit\":\"K\",\"PortLabel\":\"batteryTemperature\",\"Probing\":\"ON\"},\"batteryVoltage\":{\"Unit\":\"V\",\"PortLabel\":\"batteryVoltage\",\"Probing\":\"ON\"},\"numCycles\":{\"Unit\":\"1\",\"PortLabel\":\"numCycles\",\"Probing\":\"ON\"},\"socCell\":{\"Unit\":\"1\",\"PortLabel\":\"socCell\",\"Probing\":\"ON\"},\"socParallelAssembly\":{\"Unit\":\"1\",\"PortLabel\":\"socParallelAssembly\",\"Probing\":\"ON\"},\"vParallelAssembly\":{\"Unit\":\"V\",\"PortLabel\":\"vParallelAssembly\",\"Probing\":\"ON\"}}"
  balancingSelector1 : Selector  InputPortWidth=25  IndexOptions=Index vector (dialog)  Indices="[1  2  3  4  5]"  OutputSizes=1
  balancingSelector2 : Selector  InputPortWidth=25  IndexOptions=Index vector (dialog)  Indices="[6   7   8   9  10]"  OutputSizes=1
  balancingSelector3 : Selector  InputPortWidth=25  IndexOptions=Index vector (dialog)  Indices="[11  12  13  14  15]"  OutputSizes=1
  balancingSelector4 : Selector  InputPortWidth=25  IndexOptions=Index vector (dialog)  Indices="[16  17  18  19  20]"  OutputSizes=1
  balancingSelector5 : Selector  InputPortWidth=25  IndexOptions=Index vector (dialog)  Indices="[21  22  23  24  25]"  OutputSizes=1
  batteryCurrentMux : Mux  Inputs=5
  batteryTemperatureMux : Mux  Inputs=5
  batteryVoltageMux : Mux  Inputs=5
  numCyclesMux : Mux  Inputs=5
  socCellMux : Mux  Inputs=5
  socParallelAssemblyMux : Mux  Inputs=5
  vParallelAssemblyMux : Mux  Inputs=5
  + : PMIOPort  Side=Left
  - : PMIOPort  Port=2  Side=Right
  ClntH : PMIOPort  Port=3  Side=Right  ConnectionType=Connection: foundation.thermal.thermal
  batteryCurrent : Outport
  batteryTemperature : Outport  Port=2
  batteryVoltage : Outport  Port=3
  numCycles : Outport  Port=4
  socCell : Outport  Port=5
  socParallelAssembly : Outport  Port=6
  vParallelAssembly : Outport  Port=7
  wires:
  EVModule_outputs/1 -> [batteryCurrent1]
  batteryCurrentMux/1 -> batteryCurrent/1
  [batteryCurrent1] -> batteryCurrentMux/1
  EVModule_outputs/2 -> [batteryTemperature1]
  batteryTemperatureMux/1 -> batteryTemperature/1
  [batteryTemperature1] -> batteryTemperatureMux/1
  EVModule_outputs/3 -> [batteryVoltage1]
  batteryVoltageMux/1 -> batteryVoltage/1
  [batteryVoltage1] -> batteryVoltageMux/1
  EVModule_outputs/4 -> [numCycles1]
  numCyclesMux/1 -> numCycles/1
  [numCycles1] -> numCyclesMux/1
  EVModule_outputs/5 -> [socCell1]
  socCellMux/1 -> socCell/1
  [socCell1] -> socCellMux/1
  EVModule_outputs/6 -> [socParallelAssembly1]
  socParallelAssemblyMux/1 -> socParallelAssembly/1
  [socParallelAssembly1] -> socParallelAssemblyMux/1
  EVModule_outputs/7 -> [vParallelAssembly1]
  vParallelAssemblyMux/1 -> vParallelAssembly/1
  [vParallelAssembly1] -> vParallelAssemblyMux/1
  Module2_outputs/1 -> [batteryCurrent2]
  [batteryCurrent2] -> batteryCurrentMux/2
  Module2_outputs/2 -> [batteryTemperature2]
  [batteryTemperature2] -> batteryTemperatureMux/2
  Module2_outputs/3 -> [batteryVoltage2]
  [batteryVoltage2] -> batteryVoltageMux/2
  Module2_outputs/4 -> [numCycles2]
  [numCycles2] -> numCyclesMux/2
  Module2_outputs/5 -> [socCell2]
  [socCell2] -> socCellMux/2
  Module2_outputs/6 -> [socParallelAssembly2]
  [socParallelAssembly2] -> socParallelAssemblyMux/2
  Module2_outputs/7 -> [vParallelAssembly2]
  [vParallelAssembly2] -> vParallelAssemblyMux/2
  Module3_outputs/1 -> [batteryCurrent3]
  [batteryCurrent3] -> batteryCurrentMux/3
  Module3_outputs/2 -> [batteryTemperature3]
  [batteryTemperature3] -> batteryTemperatureMux/3
  Module3_outputs/3 -> [batteryVoltage3]
  [batteryVoltage3] -> batteryVoltageMux/3
  Module3_outputs/4 -> [numCycles3]
  [numCycles3] -> numCyclesMux/3
  Module3_outputs/5 -> [socCell3]
  [socCell3] -> socCellMux/3
  Module3_outputs/6 -> [socParallelAssembly3]
  [socParallelAssembly3] -> socParallelAssemblyMux/3
  Module3_outputs/7 -> [vParallelAssembly3]
  [vParallelAssembly3] -> vParallelAssemblyMux/3
  Module4_outputs/1 -> [batteryCurrent4]
  [batteryCurrent4] -> batteryCurrentMux/4
  Module4_outputs/2 -> [batteryTemperature4]
  [batteryTemperature4] -> batteryTemperatureMux/4
  Module4_outputs/3 -> [batteryVoltage4]
  [batteryVoltage4] -> batteryVoltageMux/4
  Module4_outputs/4 -> [numCycles4]
  [numCycles4] -> numCyclesMux/4
  Module4_outputs/5 -> [socCell4]
  [socCell4] -> socCellMux/4
  Module4_outputs/6 -> [socParallelAssembly4]
  [socParallelAssembly4] -> socParallelAssemblyMux/4
  Module4_outputs/7 -> [vParallelAssembly4]
  [vParallelAssembly4] -> vParallelAssemblyMux/4
  Module5_outputs/1 -> [batteryCurrent5]
  [batteryCurrent5] -> batteryCurrentMux/5
  Module5_outputs/2 -> [batteryTemperature5]
  [batteryTemperature5] -> batteryTemperatureMux/5
  Module5_outputs/3 -> [batteryVoltage5]
  [batteryVoltage5] -> batteryVoltageMux/5
  Module5_outputs/4 -> [numCycles5]
  [numCycles5] -> numCyclesMux/5
  Module5_outputs/5 -> [socCell5]
  [socCell5] -> socCellMux/5
  Module5_outputs/6 -> [socParallelAssembly5]
  [socParallelAssembly5] -> socParallelAssemblyMux/5
  Module5_outputs/7 -> [vParallelAssembly5]
  [vParallelAssembly5] -> vParallelAssemblyMux/5
  [balancing1] -> Converter1/1
  balancing/1 -> balancingSelector1/1, balancingSelector2/1, balancingSelector3/1, balancingSelector4/1, balancingSelector5/1
  balancingSelector1/1 -> [balancing1]
  [balancing2] -> Converter2/1
  balancingSelector2/1 -> [balancing2]
  [balancing3] -> Converter3/1
  balancingSelector3/1 -> [balancing3]
  [balancing4] -> Converter4/1
  balancingSelector4/1 -> [balancing4]
  [balancing5] -> Converter5/1
  balancingSelector5/1 -> [balancing5]
  connections:
  Module2/LConn3 -- EVModule/RConn1
  Module3/LConn3 -- Module2/RConn1
  Module4/LConn3 -- Module3/RConn1
  Module5/LConn3 -- Module4/RConn1
  EVModule/LConn3 -- +/RConn1
  Module5/RConn1 -- -/RConn1
  Converter1/RConn1 -- EVModule/LConn1
  Converter2/RConn1 -- Module2/LConn1
  Converter3/RConn1 -- Module3/LConn1
  Converter4/RConn1 -- Module4/LConn1
  Converter5/RConn1 -- Module5/LConn1
  ClntH_To_1/LConn1 -- EVModule/LConn2
  ClntH_From_1/LConn1 -- ClntH_From_2/LConn1 -- ClntH_From_3/LConn1 -- ClntH_From_4/LConn1 -- ClntH/RConn1 -- ClntH_From_5/LConn1
  ClntH_To_2/LConn1 -- Module2/LConn2
  ClntH_To_3/LConn1 -- Module3/LConn2
  ClntH_To_4/LConn1 -- Module4/LConn2
  ClntH_To_5/LConn1 -- Module5/LConn2
